simulink library "wpnav_lib"  (R2018b)
settings: Solver=VariableStepAuto  StartTime=0.0  StopTime=10.0  RelTol=1e-3
undefined symbols (not defined in the file or in its folder): ap, wpnav
libraries: filters_lib x3, simulink x1
settings Model: Creator=fabian  LastModifiedBy=yannic

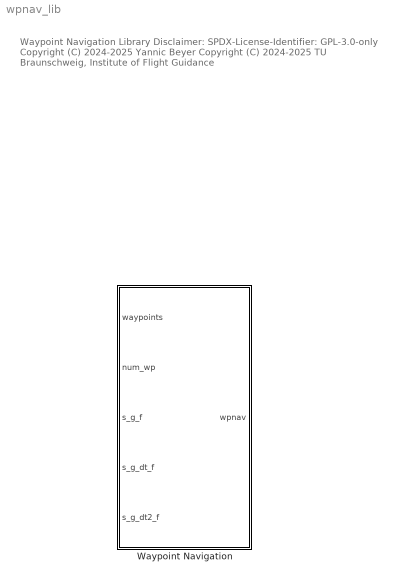
== system wpnav_lib ==
  note: Waypoint Navigation Library
      |
      | Disclaimer:
      | SPDX-License-Identifier: GPL-3.0-only
      |
      | Copyright (C) 2024-2025 Yannic Beyer
      | Copyright (C) 2024-2025 TU Braunschweig, Institute of Flight Guidance
  Waypoint Navigation : Subsystem  mask{wpnav=wpnav, T_inner_loop=0.1, is_enable_checked=off, states_when_enabling=held, mask_expr_handling_config=default}
      mask prompts: wpnav "Waypoint navigation parameters struct"; T_inner_loop "Inner loop time constant, in s"; is_enable_checked "Activate "Enabled Subsystem""; states_when_enabling "States when enabling:"
      mask init:
      | cntrlBlockInit(is_enable_checked,states_when_enabling);
      | 
      | maskExprHandling(gcbh, mask_expr_handling_config);
      mask TypeOptions states_when_enabling: held | reset
      mask TypeOptions mask_expr_handling_config: default | passthrough (tunable)
      mask DialogControl Container4 Prompt: Enable / Disable
      mask DialogControl CodeGenerationSettings Prompt: Code Generation Settings
      mask DialogControl maskExprHandlingText Prompt: Mask expression handling
      mask DialogControl maskExprHandlingReadme Prompt: README

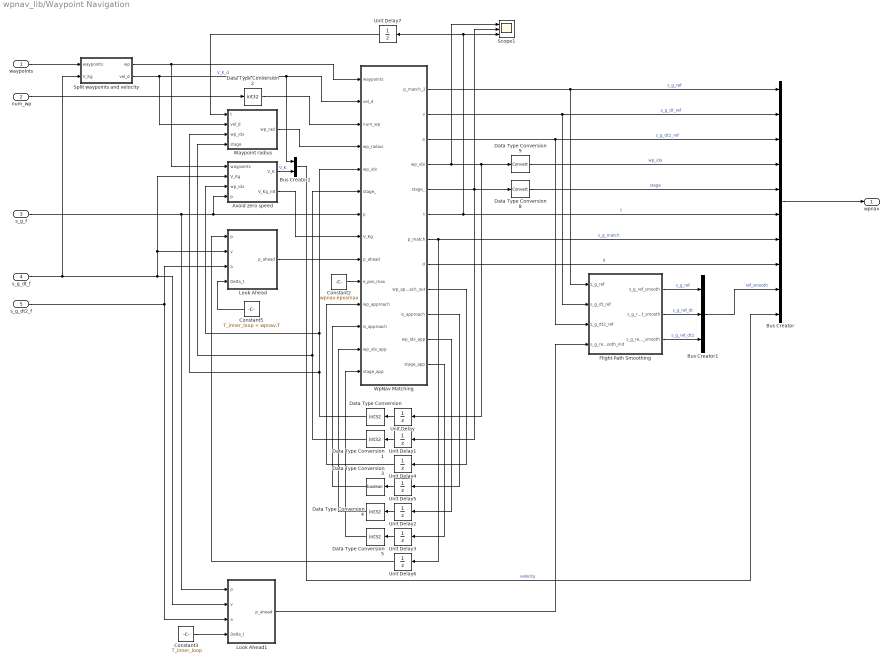
== system wpnav_lib/Waypoint Navigation ==
  waypoints : Inport
  num_wp : Inport  Port=2
  s_g_f : Inport  Port=3
  s_g_dt_f : Inport  Port=4
  s_g_dt2_f : Inport  Port=5
  Avoid zero speed : MATLAB Function  TreatAsAtomicUnit=on
  Bus Creator : BusCreator  Inputs=10
  Bus Creator1 : BusCreator  Inputs=3
  Bus Creator2 : BusCreator  Inputs=2
  Constant2 : Constant  Value=wpnav.eposmax
  Constant3 : Constant  Value=T_inner_loop
  Constant5 : Constant  Value=T_inner_loop + wpnav.T
  Data Type Conversion{,1..2,4..5} (5 alike) : DataTypeConversion  OutDataTypeStr=int32
  Data Type Conversion3 : DataTypeConversion  OutDataTypeStr=boolean
  Data Type Conversion8 : DataTypeConversion
  Data Type Conversion9 : DataTypeConversion
  Flight Path Smoothing : Subsystem
  Look Ahead : MATLAB Function  TreatAsAtomicUnit=on
  Look Ahead1 : MATLAB Function  TreatAsAtomicUnit=on
  Scope1 : Scope  NumInputPorts=3
  Split waypoints and velocity : MATLAB Function  TreatAsAtomicUnit=on
  Unit Delay{,1,6..7} (4 alike) : UnitDelay  InitialCondition=1  SampleTime=-1
  Unit Delay2 : UnitDelay  InitialCondition=2  SampleTime=-1
  Unit Delay3 : UnitDelay  SampleTime=-1
  Unit Delay4 : UnitDelay  InitialCondition=zeros(3,5)  SampleTime=-1
  Unit Delay5 : UnitDelay  SampleTime=-1
  Waypoint radius : Subsystem
  WpNav Matching : MATLAB Function  TreatAsAtomicUnit=on
  wpnav : Outport
  wires:
  Bus Creator2/1 -> Bus Creator/10  "velocity"
  Avoid zero speed/1(V_K) -> Bus Creator2/2  "V_K"
  Bus Creator1/1 -> Bus Creator/9  "ref_smooth"
  Flight Path Smoothing/3(s_g_ref_dt2_smooth) -> Bus Creator1/3  "s_g_ref_dt2"
  Flight Path Smoothing/2(s_g_ref_dt_smooth) -> Bus Creator1/2  "s_g_ref_dt"
  Flight Path Smoothing/1(s_g_ref_smooth) -> Bus Creator1/1  "s_g_ref"
  Look Ahead1/1(p_ahead) -> Flight Path Smoothing/4(s_g_ref_smooth_init)
  Split waypoints and velocity/1(wp) -> Avoid zero speed/1(waypoints), WpNav Matching/1(waypoints)
  Waypoint radius/1(wp_rad) -> WpNav Matching/4(wp_radius)
  Unit Delay7/1 -> Waypoint radius/1(t)
  Avoid zero speed/2(V_Kg_n0) -> WpNav Matching/8(V_Kg)
  s_g_dt_f/1 -> Split waypoints and velocity/2(V_Kg), Avoid zero speed/2(V_Kg), Look Ahead/2(v), Look Ahead1/2(v)
  Split waypoints and velocity/2(vel_d) -> WpNav Matching/2(vel_d), Bus Creator2/1, Waypoint radius/2(vel_d)  "V_K_d"
  Unit Delay4/1 -> WpNav Matching/11(wp_approach)
  WpNav Matching/12(stage_app) -> Unit Delay3/1
  WpNav Matching/11(wp_idx_app) -> Unit Delay2/1
  WpNav Matching/10(is_approach) -> Unit Delay5/1
  WpNav Matching/5(stage_) -> Scope1/2, Data Type Conversion8/1, Unit Delay1/1
  waypoints/1 -> Split waypoints and velocity/1(waypoints)
  Look Ahead/1(p_ahead) -> WpNav Matching/9(p_ahead)
  Data Type Conversion2/1 -> WpNav Matching/3(num_wp)
  Data Type Conversion5/1 -> WpNav Matching/14("stage_app ")
  Data Type Conversion4/1 -> WpNav Matching/13("wp_idx_app ")
  Data Type Conversion3/1 -> WpNav Matching/12("is_approach ")
  Data Type Conversion1/1 -> WpNav Matching/6("stage_ "), Waypoint radius/4(stage)
  Data Type Conversion/1 -> Avoid zero speed/3(wp_idx), WpNav Matching/5("wp_idx "), Waypoint radius/3(wp_idx)
  Constant2/1 -> WpNav Matching/10(e_pos_max)
  Unit Delay5/1 -> Data Type Conversion3/1
  WpNav Matching/9(wp_approach_out) -> Unit Delay4/1
  Unit Delay3/1 -> Data Type Conversion5/1
  Unit Delay2/1 -> Data Type Conversion4/1
  num_wp/1 -> Data Type Conversion2/1
  Unit Delay1/1 -> Data Type Conversion1/1
  Unit Delay/1 -> Data Type Conversion/1
  Constant5/1 -> Look Ahead/4(Delta_t)
  WpNav Matching/8(d) -> Bus Creator/8  "d"
  WpNav Matching/6(t) -> Bus Creator/6, Unit Delay7/1, Scope1/3  "t"
  WpNav Matching/3(a) -> Flight Path Smoothing/3(s_g_dt2_ref), Bus Creator/3  "s_g_dt2_ref"
  s_g_f/1 -> Look Ahead1/1(p), Avoid zero speed/4(p), WpNav Matching/7(p)
  WpNav Matching/1(p_match_2) -> Flight Path Smoothing/1(s_g_ref), Bus Creator/1  "s_g_ref"
  s_g_dt2_f/1 -> Look Ahead/3(a), Look Ahead1/3(a)
  WpNav Matching/4(wp_idx) -> Scope1/1, Data Type Conversion9/1, Unit Delay/1
  Bus Creator/1 -> wpnav/1
  WpNav Matching/7(p_match) -> Bus Creator/7, Unit Delay6/1  "s_g_match"
  WpNav Matching/2(v) -> Flight Path Smoothing/2(s_g_dt_ref), Bus Creator/2  "s_g_dt_ref"
  Constant3/1 -> Look Ahead1/4(Delta_t)
  Data Type Conversion8/1 -> Bus Creator/5  "stage"
  Data Type Conversion9/1 -> Bus Creator/4  "wp_idx"
  Unit Delay6/1 -> Look Ahead/1(p)

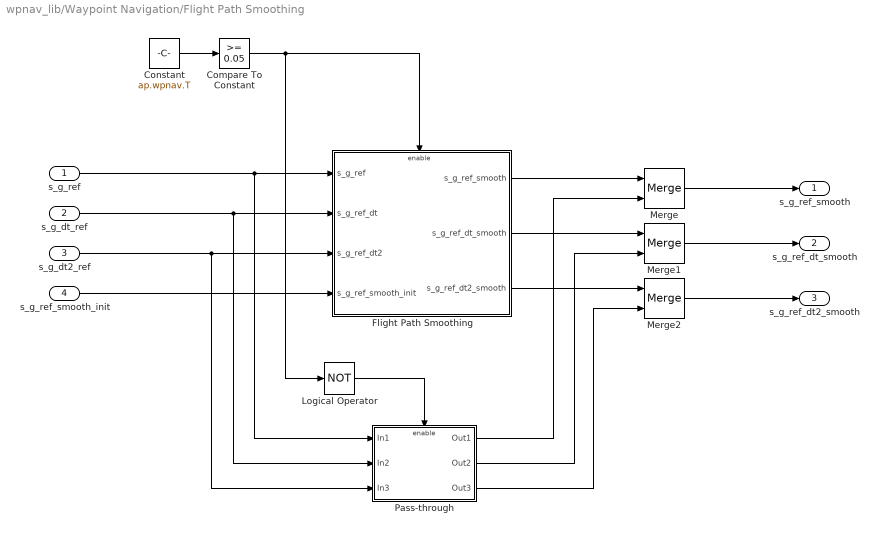
== system wpnav_lib/Waypoint Navigation/Flight Path Smoothing ==
  s_g_ref : Inport
  s_g_dt_ref : Inport  Port=2
  s_g_dt2_ref : Inport  Port=3
  s_g_ref_smooth_init : Inport  Port=4
  Compare To Constant : simulink/Logic and Bit Operations/Compare To Constant  relop=>=  const=0.05  OutDataTypeStr=boolean
  Constant : Constant  Value=ap.wpnav.T
  Flight Path Smoothing : Subsystem
  Logical Operator : Logic  Operator=NOT  AllPortsSameDT=off  OutDataTypeStr=boolean
  Merge : Merge
  Merge1 : Merge
  Merge2 : Merge
  Pass-through : Subsystem
  s_g_ref_smooth : Outport
  s_g_ref_dt_smooth : Outport  Port=2
  s_g_ref_dt2_smooth : Outport  Port=3
  wires:
  Logical Operator/1 -> Pass-through/Enable
  Pass-through/3(Out3) -> Merge2/2
  Pass-through/2(Out2) -> Merge1/2
  Pass-through/1(Out1) -> Merge/2
  Merge2/1 -> s_g_ref_dt2_smooth/1
  Merge1/1 -> s_g_ref_dt_smooth/1
  Merge/1 -> s_g_ref_smooth/1
  Flight Path Smoothing/3(s_g_ref_dt2_smooth) -> Merge2/1
  Flight Path Smoothing/2(s_g_ref_dt_smooth) -> Merge1/1
  s_g_ref/1 -> Pass-through/1(In1), Flight Path Smoothing/1(s_g_ref)
  s_g_dt2_ref/1 -> Pass-through/3(In3), Flight Path Smoothing/3(s_g_ref_dt2)
  s_g_dt_ref/1 -> Pass-through/2(In2), Flight Path Smoothing/2(s_g_ref_dt)
  Compare To Constant/1 -> Flight Path Smoothing/Enable, Logical Operator/1
  Flight Path Smoothing/1(s_g_ref_smooth) -> Merge/1
  s_g_ref_smooth_init/1 -> Flight Path Smoothing/4(s_g_ref_smooth_init)
  Constant/1 -> Compare To Constant/1

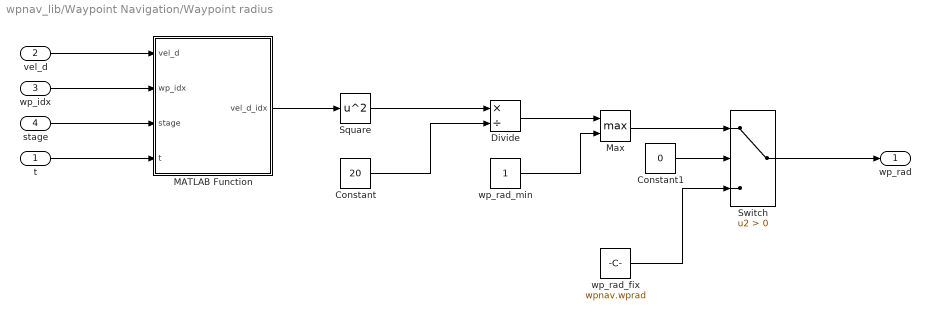
== system wpnav_lib/Waypoint Navigation/Waypoint radius ==
  t : Inport
  vel_d : Inport  Port=2
  wp_idx : Inport  Port=3
  stage : Inport  Port=4
  Constant : Constant  Value=20
  Constant1 : Constant  Value=0
  Divide : Product  Inputs=*/
  MATLAB Function : MATLAB Function  TreatAsAtomicUnit=on
  Max : MinMax  Function=max  Inputs=2
  Square : Math  Operator=square  SaturateOnIntegerOverflow=on
  Switch : Switch  Criteria=u2 > Threshold
  wp_rad_fix : Constant  Value=wpnav.wprad
  wp_rad_min : Constant
  wp_rad : Outport
  wires:
  wp_rad_fix/1 -> Switch/3
  Constant1/1 -> Switch/2
  Switch/1 -> wp_rad/1
  Max/1 -> Switch/1
  Constant/1 -> Divide/2
  wp_idx/1 -> MATLAB Function/2(wp_idx)
  t/1 -> MATLAB Function/4(t)
  stage/1 -> MATLAB Function/3(stage)
  wp_rad_min/1 -> Max/2
  vel_d/1 -> MATLAB Function/1(vel_d)
  MATLAB Function/1(vel_d_idx) -> Square/1
  Square/1 -> Divide/1
  Divide/1 -> Max/1

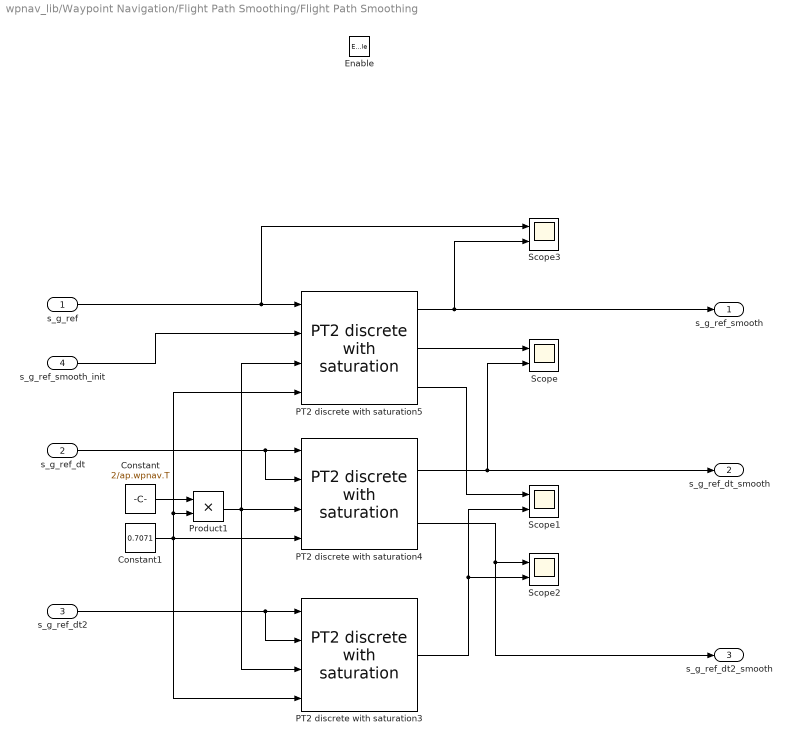
== system wpnav_lib/Waypoint Navigation/Flight Path Smoothing/Flight Path Smoothing ==
  s_g_ref : Inport
  s_g_ref_dt : Inport  Port=2
  s_g_ref_dt2 : Inport  Port=3
  s_g_ref_smooth_init : Inport  Port=4
  Enable : EnablePort  StatesWhenEnabling=reset
  Constant : Constant  Value=2/ap.wpnav.T
  Constant1 : Constant  Value=0.7071
  PT2 discrete with saturation3 : filters_lib/PT2 discrete with saturation  param_src=external  omega=1  d=1  x_max=inf  x_min=-inf  x_dt_max=inf  x_dt_min=-inf  x_dt2_max=inf  x_dt2_min=-inf  y_0_src=external  x_init=0  y_dt_0_src=internal  x_dt_init=0  is_y_dt_checked=off  is_y_dt2_checked=off  is_external_reset_checked=off  mask_expr_handling_config=default
      settings: SourceProductName=LADAC
  PT2 discrete with saturation4 : filters_lib/PT2 discrete with saturation  param_src=external  omega=1  d=1  x_max=inf  x_min=-inf  x_dt_max=inf  x_dt_min=-inf  x_dt2_max=inf  x_dt2_min=-inf  y_0_src=external  x_init=0  y_dt_0_src=internal  x_dt_init=0  is_y_dt_checked=on  is_y_dt2_checked=off  is_external_reset_checked=off  mask_expr_handling_config=default
      settings: SourceProductName=LADAC
  PT2 discrete with saturation5 : filters_lib/PT2 discrete with saturation  param_src=external  omega=1  d=1  x_max=inf  x_min=-inf  x_dt_max=inf  x_dt_min=-inf  x_dt2_max=inf  x_dt2_min=-inf  y_0_src=external  x_init=0  y_dt_0_src=internal  x_dt_init=0  is_y_dt_checked=on  is_y_dt2_checked=on  is_external_reset_checked=off  mask_expr_handling_config=default
      settings: SourceProductName=LADAC
  Product1 : Product
  Scope{,1..3} (4 alike) : Scope  NumInputPorts=2
  s_g_ref_smooth : Outport
  s_g_ref_dt_smooth : Outport  Port=2
  s_g_ref_dt2_smooth : Outport  Port=3
  wires:
  Product1/1 -> PT2 discrete with saturation4/3, PT2 discrete with saturation3/3, PT2 discrete with saturation5/3
  Constant1/1 -> PT2 discrete with saturation4/4, PT2 discrete with saturation3/4, Product1/2, PT2 discrete with saturation5/4
  Constant/1 -> Product1/1
  PT2 discrete with saturation4/1 -> s_g_ref_dt_smooth/1, Scope/2
  s_g_ref_dt/1 -> PT2 discrete with saturation4/1, PT2 discrete with saturation4/2
  PT2 discrete with saturation4/2 -> Scope2/1, s_g_ref_dt2_smooth/1
  PT2 discrete with saturation5/3 -> Scope1/1
  PT2 discrete with saturation5/2 -> Scope/1
  s_g_ref_dt2/1 -> PT2 discrete with saturation3/1, PT2 discrete with saturation3/2
  PT2 discrete with saturation3/1 -> Scope2/2, Scope1/2
  PT2 discrete with saturation5/1 -> Scope3/2, s_g_ref_smooth/1
  s_g_ref/1 -> Scope3/1, PT2 discrete with saturation5/1
  s_g_ref_smooth_init/1 -> PT2 discrete with saturation5/2

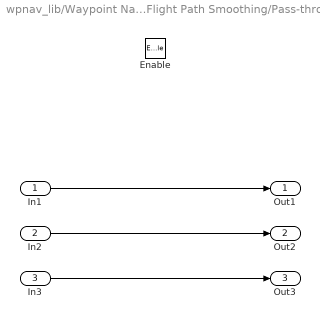
== system wpnav_lib/Waypoint Navigation/Flight Path Smoothing/Pass-through ==
  In1 : Inport
  In2 : Inport  Port=2
  In3 : Inport  Port=3
  Enable : EnablePort
  Out1 : Outport
  Out2 : Outport  Port=2
  Out3 : Outport  Port=3
  wires:
  In3/1 -> Out3/1
  In2/1 -> Out2/1
  In1/1 -> Out1/1

== matlab function wpnav_lib/Waypoint Navigation/Avoid zero speed ==
  data: V_K output; waypoints input; V_Kg input; V_Kg_n0 output; wp_idx input; p input
function [V_K,V_Kg_n0] = fcn(waypoints,V_Kg,wp_idx,p)
V_K = norm(V_Kg,2);
V_Kg_n0 = V_Kg;
if V_K < 0.3
    direction = waypoints(:,wp_idx) - p;
    direction = divideFinite(direction,norm(direction,2));
    V_Kg_n0(:) = 0.3 *  direction;
end
end

== matlab function wpnav_lib/Waypoint Navigation/Look Ahead ==
  data: p input; p_ahead output; v input; a input; Delta_t input
function p_ahead = fcn(p,v,a,Delta_t)
p_ahead = p + v*Delta_t + 0.5*a*Delta_t*Delta_t;
end

== matlab function wpnav_lib/Waypoint Navigation/Look Ahead1 ==
  data: p input; p_ahead output; v input; a input; Delta_t input
function p_ahead = fcn(p,v,a,Delta_t)

p_ahead = p + v*Delta_t + 0.5*a*Delta_t*Delta_t;

end

== matlab function wpnav_lib/Waypoint Navigation/Split waypoints and velocity ==
  data: waypoints input; wp output; vel_d output; V_Kg input
function [wp,vel_d] = fcn(waypoints, V_Kg)
if size(waypoints,2) < 1
    wp = zeros(3,2,class(waypoints));
elseif size(waypoints,2) < 2
    wp = [waypoints(1:3,:),zeros(3,1,class(waypoints))];
else
    wp = waypoints(1:3,:);
end
if size(waypoints,1)<4
    vel_d = repmat(norm(V_Kg),1,size(waypoints,2));
else
    vel_d = waypoints(4,:);
end
end

== matlab function wpnav_lib/Waypoint Navigation/Waypoint radius/MATLAB Function ==
  data: vel_d input; vel_d_idx output; wp_idx input; stage input; t input
function vel_d_idx = fcn(vel_d, wp_idx, stage, t)
if wp_idx == 1
    vel_d_prev = vel_d(end);
else
    vel_d_prev = vel_d(wp_idx-1);
end
if stage == 0
    vel_d_idx = vel_d_prev;
else
    vel_d_idx = vel_d_prev + (vel_d(wp_idx)-vel_d_prev)*sqrtReal(t);
end
end

== matlab function wpnav_lib/Waypoint Navigation/WpNav Matching ==
  data: waypoints input; vel_d input; p_match_2 output; num_wp input; wp_radius input; wp_idx input; stage_ input; p input; V_Kg input; p_ahead input; e_pos_max input; wp_approach input; is_approach input; wp_idx_app input; stage_app input; v output; a output; wp_idx output; stage_ output; t output; p_match output; d output; wp_approach_out output; is_approach output; wp_idx_app output; stage_app output
function [p_match_2,v,a,wp_idx,stage_,t,p_match,d,wp_approach_out,is_approach,wp_idx_app,stage_app] = ...
    wpnavMatchSim(waypoints, vel_d, num_wp, wp_radius, wp_idx, stage_, p, V_Kg, p_ahead, ...
    e_pos_max, wp_approach, is_approach, wp_idx_app, stage_app )

a = zeros(3,1,superiorfloat(waypoints));
v = zeros(3,1,superiorfloat(waypoints));
% Re-use of wp_approach causes data type error in the first run in
% Simulink. That is why a new variable is used.
wp_approach_out = zeros(3,5,superiorfloat(waypoints));
wp_approach_out(:) = wp_approach;

num_wp = max(num_wp,2);

if is_approach
    [p_match,wp_idx_app,stage_app,t,d] = wpnavMatch(wp_approach_out,wp_radius,wp_idx_app,stage_app,p);
    [p_match_2,wp_idx_app_2,stage_app_2,t_2,d_2] = wpnavMatch(wp_approach_out,wp_radius,wp_idx_app,stage_app,p_ahead);
    stage_2 = stage_;
    wp_idx_2 = wp_idx;
    stage_tmp = stage_;
    wp_idx_tmp = wp_idx;
else
    [p_match,wp_idx_tmp,stage_tmp,t,d] = wpnavMatch(waypoints(:,1:num_wp),wp_radius,wp_idx,stage_,p);
    [p_match_2,wp_idx_2,stage_2,t_2,d_2] = wpnavMatch(waypoints(:,1:num_wp),wp_radius,wp_idx,stage_,p_ahead);
    stage_app_2 = stage_app;
    wp_idx_app_2 = wp_idx_app;
end


e_pos = norm(p_match-p,2);
if e_pos > e_pos_max
    dir_next_wp = waypoints(:,wp_idx) - p;
    dist_next_wp = norm( dir_next_wp );
    flight_dir = divideFinite( V_Kg, norm(V_Kg,2) );
    angle_next_wp = acosReal( divideFinite( dot( dir_next_wp, flight_dir ), norm(dir_next_wp,2)*norm(flight_dir,2) ) );
    if angle_next_wp < 0.5 && dist_next_wp < wp_radius
        dist_app_wp = 0.5 * dist_next_wp;
    else
        dist_app_wp = 1.2*wp_radius;
    end
    wp_approach_out(:,1) = p - flight_dir * 1 * dist_app_wp;
    wp_approach_out(:,2) = p + flight_dir * 1 * dist_app_wp;
    wp_approach_out(:,3) = waypoints(:,wp_idx);
    if wp_idx == num_wp-1
        wp_approach_out(:,4) = waypoints(:,wp_idx);
        wp_approach_out(:,5) = waypoints(:,1);
    elseif wp_idx == num_wp
        wp_approach_out(:,4) = waypoints(:,1);
        wp_approach_out(:,5) = waypoints(:,2);
    else
        wp_approach_out(:,4) = waypoints(:,wp_idx+1);
        wp_approach_out(:,5) = waypoints(:,wp_idx+2);
    end
    is_approach(:) = 1;
    wp_idx_app(:) = 2;
    stage_app(:) = 1;
    [p_match,wp_idx_app,stage_app,t,d] = wpnavMatch(wp_approach_out,wp_radius,wp_idx_app,stage_app,p);
    [p_match_2,wp_idx_app_2,stage_app_2,t_2,d_2] = wpnavMatch(wp_approach_out,wp_radius,wp_idx_app,stage_app,p_ahead);
    stage_2 = stage_;
    wp_idx_2 = wp_idx;
else
    wp_idx = wp_idx_tmp;
    stage_ = stage_tmp;
end
if (wp_idx_app == 4 && stage_app == 1) || wp_idx_app == 5
    wp_idx_app(:) = 2;
    is_approach(:) = 0;
    wp_idx_new = wp_idx + 1;
    stage_(:) = 1;
    [p_match,wp_idx,stage_,t,d] = wpnavMatch(waypoints(:,1:num_wp),wp_radius,wp_idx_new,stage_,p);
    % If there is no straight line, avoid duplicate wp_idx increment
    if wp_idx ~= wp_idx_new
        [p_match,wp_idx,stage_,t,d] = wpnavMatch(waypoints(:,1:num_wp),wp_radius,wp_idx_new-1,stage_,p);
    end
    [p_match_2,wp_idx_2,stage_2,t_2,d_2] = wpnavMatch(waypoints(:,1:num_wp),wp_radius,wp_idx,stage_,p_ahead);
    stage_app_2 = stage_app;
    wp_idx_app_2 = wp_idx_app;
end


prev_wp_idx = wp_idx-1;
if prev_wp_idx <= 0
    prev_wp_idx(:) = num_wp;
end
if stage_ == 0
    V_K = vel_d(prev_wp_idx);
else
    V_K = vel_d(prev_wp_idx) + (vel_d(wp_idx)-vel_d(prev_wp_idx)) * t; %sqrtReal(t);
end

if (stage_2 == 0 && ~is_approach) || (stage_app_2 == 0 && is_approach)
    if ~is_approach
        if wp_idx_2 > 2
            waypoints3x3 = waypoints(:,wp_idx_2-2:wp_idx_2);
        elseif wp_idx_2 == 2
            waypoints3x3 = waypoints(:,[num_wp,1,2]);
        else
            waypoints3x3 = waypoints(:,[num_wp-1,num_wp,1]);
        end
    else
        if wp_idx_app_2 > 2
            waypoints3x3 = wp_approach_out(:,wp_idx_app_2-2:wp_idx_app_2);
        elseif wp_idx_app_2 == 2
            waypoints3x3 = wp_approach_out(:,[end,1,2]);
        else
            waypoints3x3 = wp_approach_out(:,[end-1,end,1]);
        end
    end
    circ_seg = wpnavCircSeg(waypoints3x3,wp_radius);
    v(:) = wpnavCircSegGetVel(circ_seg,t_2,V_K);
    a(:) = wpnavCircSegGetAcc(circ_seg,t_2,V_K);
% elseif (stage_2 == 1 && ~is_approach) || (stage_app_2 == 1 && is_approach)
else
    if ~is_approach
        if wp_idx_2 > 1
            wp1 = waypoints(:,wp_idx_2-1);
            wp2 = waypoints(:,wp_idx_2);
        else
            wp1 = waypoints(:,num_wp);
            wp2 = waypoints(:,1);
        end
    else
        wp1 = wp_approach_out(:,wp_idx_app_2-1);
        wp2 = wp_approach_out(:,wp_idx_app_2);
    end
    v(:) = wpnavLineGetVel(wp1,wp2,V_K);
end

end
